simulink model "pend_lin_samir"  (R2017b)
settings: Solver=VariableStepAuto  StartTime=0.0  StopTime=500  RelTol=1e-3
values from neighbouring files (symbols this model uses):
  Jm = 3.1e-7    (= 3.1e-07)    [pend.m]
  Jp = 1774.274e-6    (= 0.001774274)    [pend.m]
  kd = 2.5    [pend.m]
  Kf = 7.44e-3    (= 0.00744)    [pend.m]
  ki = 10    [pend.m]
  kp = 5    [pend.m]
  La = 35e-6    (= 3.5e-05)    [pend.m]
  lb = 141.451e-3    (= 0.141451)    [pend.m]
  M = 879.5e-3    (= 0.8795)    [pend.m]
  m = 135.4e-3    (= 0.1354)    [pend.m]
  p1 = 0.0035    [pend.m]
  p2 = 0.0058    [pend.m]
  Ra = 3.92    [pend.m]
  Rg = 6.35e-3    (= 0.00635)    [pend.m]
  rt = 3.2067e-04    (= 0.00032067)    [pend.m]
  tet0 = pi/3    (= 1.0471975512)    [pend.m]
settings Model: Creator=lelli  LastModifiedBy=lelli

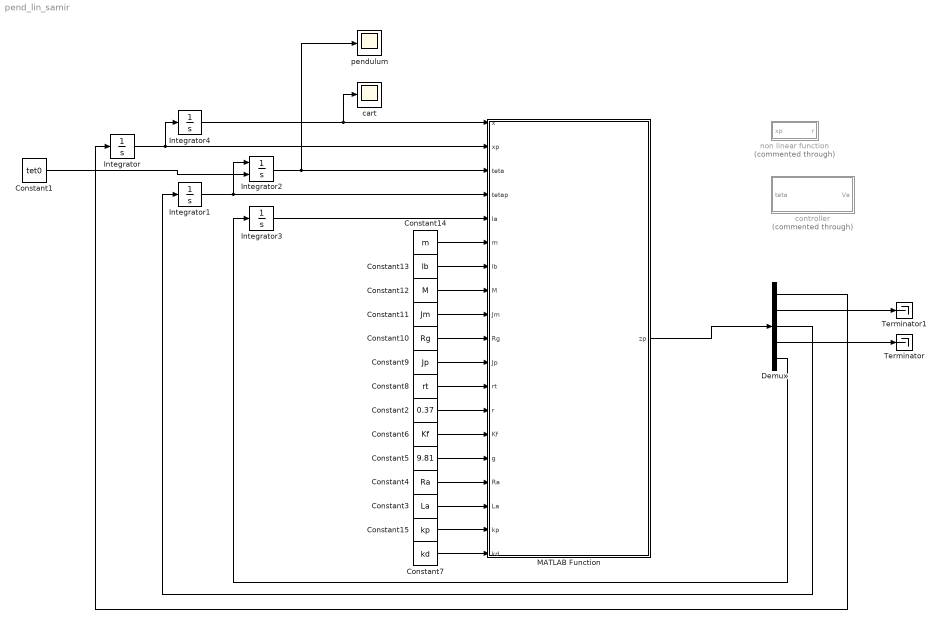
== system pend_lin_samir ==
  Constant1 : Constant  Value=tet0
  Constant10 : Constant  Value=Rg
  Constant11 : Constant  Value=Jm
  Constant12 : Constant  Value=M
  Constant13 : Constant  Value=lb
  Constant14 : Constant  Value=m
  Constant15 : Constant  Value=kp
  Constant2 : Constant  Value=0.37
  Constant3 : Constant  Value=La
  Constant4 : Constant  Value=Ra
  Constant5 : Constant  Value=9.81
  Constant6 : Constant  Value=Kf
  Constant7 : Constant  Value=kd
  Constant8 : Constant  Value=rt
  Constant9 : Constant  Value=Jp
  Demux : Demux  Outputs=5
  Integrator{,1,3..4} (4 alike) : Integrator
  Integrator2 : Integrator  InitialConditionSource=external  InitialCondition=pi/6
  MATLAB Function : MATLAB Function  TreatAsAtomicUnit=on
  Terminator : Terminator
  Terminator1 : Terminator
  cart : Scope
  controller : Subsystem  Commented=through
  non linear function : Subsystem  Commented=through
  pendulum : Scope
  wires:
  MATLAB Function/1(zp) -> Demux/1
  Demux/3 -> Integrator1/1
  Demux/1 -> Integrator/1
  Integrator1/1 -> MATLAB Function/4(tetap), Integrator2/1
  Integrator2/1 -> MATLAB Function/3(teta), pendulum/1
  Integrator3/1 -> MATLAB Function/5(Ia)
  Demux/5 -> Integrator3/1
  Constant14/1 -> MATLAB Function/6(m)
  Constant13/1 -> MATLAB Function/7(lb)
  Constant11/1 -> MATLAB Function/9(Jm)
  Constant10/1 -> MATLAB Function/10(Rg)
  Constant9/1 -> MATLAB Function/11(Jp)
  Constant8/1 -> MATLAB Function/12(rt)
  Constant6/1 -> MATLAB Function/14(Kf)
  Constant5/1 -> MATLAB Function/15(g)
  Constant4/1 -> MATLAB Function/16(Ra)
  Constant3/1 -> MATLAB Function/17(La)
  Constant12/1 -> MATLAB Function/8(M)
  Integrator4/1 -> MATLAB Function/1(x), cart/1
  Constant1/1 -> Integrator2/2
  Integrator/1 -> MATLAB Function/2(xp), Integrator4/1
  Demux/2 -> Terminator1/1
  Demux/4 -> Terminator/1
  Constant2/1 -> MATLAB Function/13(r)
  Constant7/1 -> MATLAB Function/19(kd)
  Constant15/1 -> MATLAB Function/18(kp)

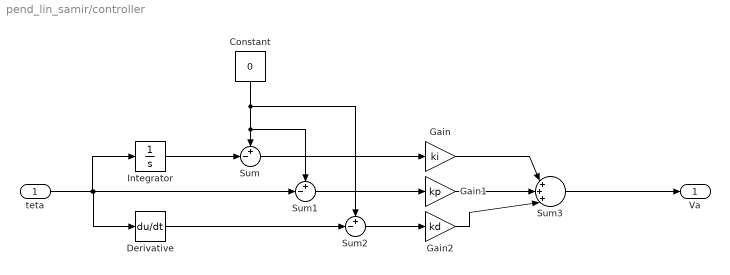
== system pend_lin_samir/controller ==
  teta : Inport
  Constant : Constant  Value=0
  Derivative : Derivative
  Gain : Gain  Gain=ki
  Gain1 : Gain  Gain=kp
  Gain2 : Gain  Gain=kd
  Integrator : Integrator
  Sum : Sum  Inputs=+-|
  Sum1 : Sum  Inputs=+-|
  Sum2 : Sum  Inputs=+-|
  Sum3 : Sum  Inputs=|+++|
  Va : Outport
  wires:
  teta/1 -> Integrator/1, Derivative/1, Sum1/2
  Constant/1 -> Sum2/1, Sum1/1, Sum/1
  Integrator/1 -> Sum/2
  Derivative/1 -> Sum2/2
  Sum/1 -> Gain/1
  Sum1/1 -> Gain1/1
  Sum2/1 -> Gain2/1
  Gain1/1 -> Sum3/2
  Gain/1 -> Sum3/1
  Gain2/1 -> Sum3/3
  Sum3/1 -> Va/1

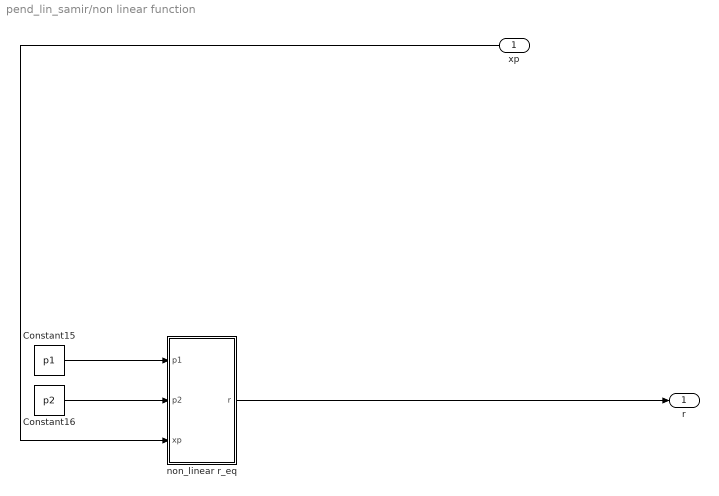
== system pend_lin_samir/non linear function ==
  xp : Inport
  Constant15 : Constant  Value=p1
  Constant16 : Constant  Value=p2
  "non_linear r_eq " : MATLAB Function  TreatAsAtomicUnit=on
  r : Outport
  wires:
  Constant16/1 -> "non_linear r_eq "/2(p2)
  Constant15/1 -> "non_linear r_eq "/1(p1)
  "non_linear r_eq "/1(r) -> r/1
  xp/1 -> "non_linear r_eq "/3(xp)

== matlab function pend_lin_samir/non linear function/non_linear r_eq  ==
  data: p1 input; r output; p2 input; xp input
function r  = r_eq(p1,p2,xp)
%non linear relationship between velocity and cart dumping
%p1 is the slope of linear approximation of force measured
%p2 is the intercept of linear approximation of force measured
%xp is the instantaneous velocity 
if xp>1e-10 || xp<-1e-10
    r=2*p2/pi*atan(100*xp)/xp + p1;
else
    r=2*p2/pi*100+p1;
end
end

== matlab function pend_lin_samir/MATLAB Function ==
  data: x input; xp input; zp output; teta input; tetap input; Ia input; m input; lb input; M input; Jm input; Rg input; Jp input; rt input; r input; Kf input; g input; Ra input; La input; kp input; kd input
function zp = pend_lin_sys(x,xp,teta,tetap,Ia,m,lb,M,Jm,Rg,Jp,rt,r,Kf,g,Ra,La,kp,kd)
%Va=kp*(-teta)+kd*(-tetap);
Va = 0;
z=[xp x tetap teta Ia];
z=z';
M=[M + m + Jm/Rg^2 0 m*lb 0 0; 
   0 1 0 0 0; 
   m*lb 0 Jp+m*lb^2 0 0; 
   0 0 0 1 0;
   0 0 0 0 La]; %multipling Zp
N=[-r 0 0 0 Kf/Rg;
    1 0 0 0 0;
    0 0 -rt -m*g*lb 0;
    0 0 1 0 0;
   - Kf/Rg 0 0 0 -Ra]; %multipling Z
P=[0;
   0;
   0;
   0;
   1]; % multipling Va
A=(M\N);  B=M\P;
zp = A*z + B*Va;
